simulink model "V40AeroDynamics_edit_3D"  (R2017b)
settings: Solver=VariableStepAuto  StartTime=0.0  StopTime=500  RelTol=1e-3
values from neighbouring files (symbols this model uses):
  A = [ 0        0        0        1 ... (first row only)    [LinearV40.m]
  B = [ 0         0 ... (first row only)    [LinearV40.m]
  b_ref = 5.1    [V40_CFD.mat]
  C = [1       0       0       0 ... (first row only)    [LinearV40.m]
  c_bar = 0.321    [V40_CFD.mat]
  CG_ref_x = 1.38    [V40_CFD.mat]
  CG_ref_z = 0    [V40_CFD.mat]
  CL0 = 0.3831    [V40_CFD.mat]
  Clp = -0.595    [V40_CFD.mat]
  Clr = 0.005    [V40_CFD.mat]
  Cm0 = 0.109    [V40_CFD.mat]
  Cmq = -24.09    [V40_CFD.mat]
  Cnp = 0    [V40_CFD.mat]
  Cnr = -0.023    [V40_CFD.mat]
  CX_d_ca_l =     [V40_CFD.mat]
  CX_d_ca_r =     [V40_CFD.mat]
  CX_d_ea_l =     [V40_CFD.mat]
  CX_d_ea_r =     [V40_CFD.mat]
  CX_d_r =     [V40_CFD.mat]
  D = zeros(size(C,1),2)    [LinearV40.m]
  D_CL_alpha = [-1.0711 -0.8677 -0.6557 -0.4384 -0.2189 0 0.2148 0.422 0.6186 0.8018 0.9688 1.1173 ... (17 elements, 1x17)]    [V40_CFD.mat]
  D_Cm_alpha = [0.0153 0.0193 0.0198 0.0168 0.0102 0 -0.0133 -0.0293 -0.0475 -0.0672 -0.0875 -0.1073 ... (17 elements, 1x17)]    [V40_CFD.mat]
  DCD_alpha = [0.1342 0.0942 0.065 0.0469 0.0395 0.0429 0.0567 0.0807 0.1143 0.1571 0.2086 0.2683 ... (17 elements, 1x17)]    [V40_CFD.mat]
  DCX_beta =     [V40_CFD.mat]
  g = 9.79    [trim_v40.m]    (also in trim_v40_3D.m = 9.8)
  Iv = [13.1154, 0, 0; 0, 9.9543, 0; 0, 0, 15.7149]    [trim_v40.m]    (also in trim_v40_3D.m)
  pitchTheta0 = 0.0521    [LinearV40.m]
  q0 = 0    [LinearV40.m]    (also in trim_v40.m; trim_v40_3D.m)
  rho = 1.213    [trim_v40.m]    (also in trim_v40_3D.m)
  S_ref = 1.4    [V40_CFD.mat]
  Thrust = 39.9    [LinearV40.m]    (also in trim_v40_3D.m = 64.7)
  u0 = 26.152    [LinearV40.m]    (also in trim_v40.m = Vg(1); trim_v40_3D.m = Vg(1))
  w0 = 1.231    [LinearV40.m]    (also in trim_v40.m = Vg(3); trim_v40_3D.m = Vg(3))
  x0 = 0    [LinearV40.m]    (also in trim_v40.m; trim_v40_3D.m)
  x_CG = 1.38-0.043    (= 1.337)    [trim_v40.m]    (also in trim_v40_3D.m)
  z0 = -200    [LinearV40.m]    (also in trim_v40.m; trim_v40_3D.m)
  z_CG = 0    [trim_v40.m]    (also in trim_v40_3D.m)
libraries: simulink_extras x3, shared3dof x1, aerolibasang x1, aerolibtransform2 x1
(part 1 of 2)
settings Model: Creator=ken  LastModifiedBy=ken

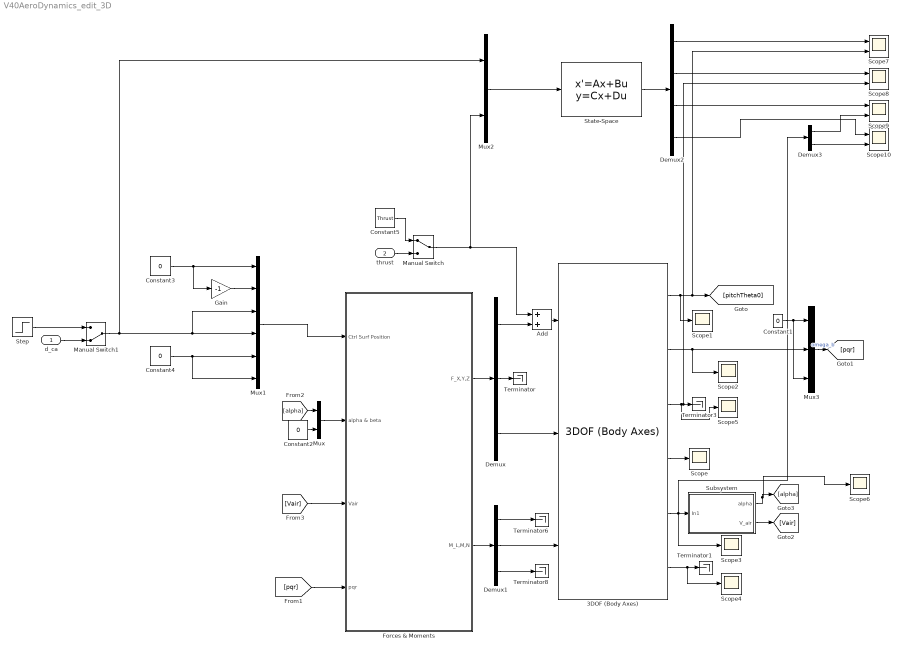
== system V40AeroDynamics_edit_3D ==
  d_ca : Inport
  thrust : Inport  Port=2
  3DOF (Body Axes) : shared3dof/3DOF (Body Axes)  units=Metric (MKS)  mtype=Fixed  v_ini=Vair0  theta_ini=pitchTheta0  alpha_ini=alpha0  q_ini=q0  pos_ini=[x0,z0]  mass=mass0  mass_e=0.5  mass_f=3.0  Iyy=Iv(2,2)  Iyy_e=0.5  Iyy_f=3.0  g_in=Internal  g=g  vre_flag=on  abi_flag=off
      settings: SourceProductName=Aerospace Blockset  SourceProductBaseCode=AE
  Add : Sum
  Constant{1..4} (4 alike) : Constant  Value=0
  Constant5 : Constant  Value=Thrust
  Demux : Demux  Outputs=3
  Demux1 : Demux  Outputs=3
  Demux2 : Demux
  Demux3 : Demux  Outputs=2
  Forces & Moments : Subsystem
  Gain : Gain  Gain=-1
  Manual Switch : ManualSwitch
  Manual Switch1 : ManualSwitch  CurrentSetting=0
  Mux : Mux  Inputs=2
  Mux1 : Mux  Inputs=6
  Mux2 : Mux  Inputs=2
  Mux3 : Mux  Inputs=3
  Scope{,1..6} (7 alike) : Scope
  Scope{7..10} (4 alike) : Scope  NumInputPorts=2
  State-Space : StateSpace  A=A  B=B  C=C  D=D  InitialCondition=[pitchTheta0 u0 w0 q0]
  Step : Step  After=5  SampleTime=0
  Subsystem : Subsystem
  Terminator{,1,3,6,8} (5 alike) : Terminator
  wires:
  Forces & Moments/2(M_L,M,N) -> Demux1/1
  Gain/1 -> Mux1/2
  Constant4/1 -> Mux1/6, Mux1/5
  Demux/2 -> Terminator/1
  Constant3/1 -> Gain/1, Mux1/1
  Demux/3 -> 3DOF (Body Axes)/2
  Manual Switch/1 -> Add/1, Mux2/2
  Demux1/3 -> Terminator8/1
  Demux1/1 -> Terminator6/1
  Forces & Moments/1(F_X,Y,Z) -> Demux/1
  Mux1/1 -> Forces & Moments/1(Ctrl Surf Position)
  Manual Switch1/1 -> Mux2/1, Mux1/3, Mux1/4
  Constant2/1 -> Mux/2
  Mux/1 -> Forces & Moments/2(alpha & beta)
  3DOF (Body Axes)/4 -> Scope/1
  3DOF (Body Axes)/3 -> Scope5/1, Scope8/2, Terminator3/1
  3DOF (Body Axes)/2 -> Scope2/1, Mux3/2
  Constant1/1 -> Mux3/3, Mux3/1
  3DOF (Body Axes)/6 -> Scope4/1, Terminator1/1
  thrust/1 -> Manual Switch/2
  Constant5/1 -> Manual Switch/1
  d_ca/1 -> Manual Switch1/2
  Step/1 -> Manual Switch1/1
  3DOF (Body Axes)/1 -> Scope1/1, Scope7/2, [pitchTheta0]
  Mux3/1 -> [pqr]  "omega_b"
  [pqr] -> Forces & Moments/4(pqr)
  3DOF (Body Axes)/5 -> Demux3/1, Scope3/1, Subsystem/1(In1)
  Subsystem/2(V_air) -> [Vair]
  Subsystem/1(alpha) -> Scope6/1, [alpha]
  [Vair] -> Forces & Moments/3(Vair)
  [alpha] -> Mux/1
  Demux1/2 -> 3DOF (Body Axes)/3
  Demux/1 -> Add/2
  Add/1 -> 3DOF (Body Axes)/1
  Mux2/1 -> State-Space/1
  State-Space/1 -> Demux2/1
  Demux2/1 -> Scope7/1
  Demux2/2 -> Scope8/1
  Demux2/3 -> Scope9/1
  Demux3/1 -> Scope9/2
  Demux2/4 -> Scope10/1
  Demux3/2 -> Scope10/2

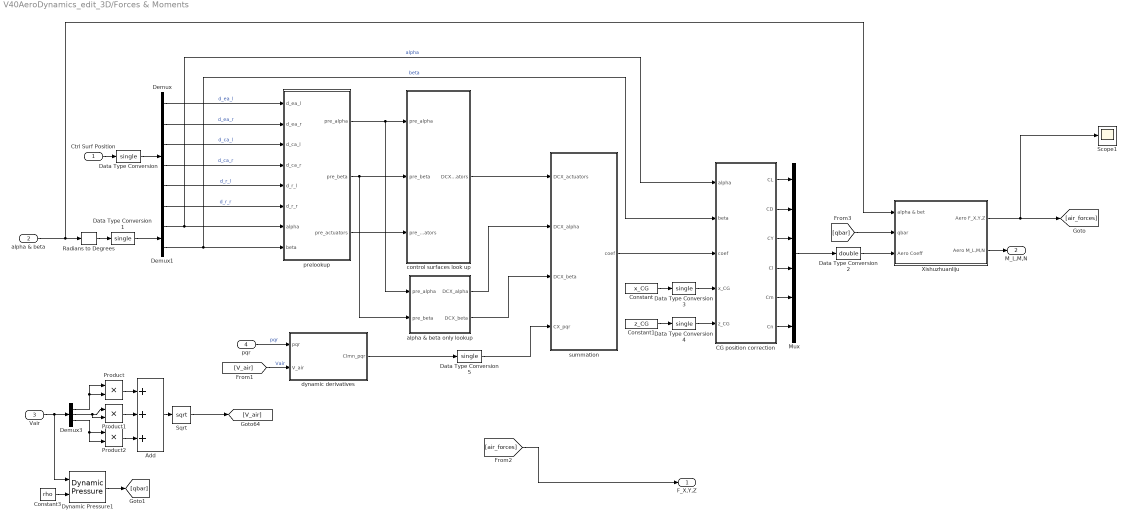
== system V40AeroDynamics_edit_3D/Forces & Moments ==
  Ctrl Surf Position : Inport
  alpha & beta : Inport  Port=2
  Vair : Inport  Port=3
  pqr : Inport  Port=4
  Add : Sum  Inputs=+++
  CG position correction : Subsystem
  Constant : Constant  Value=x_CG
  Constant1 : Constant  Value=z_CG
  Constant3 : Constant  Value=rho
  Data Type Conversion{,1,3..5} (5 alike) : DataTypeConversion  OutDataTypeStr=single
  Data Type Conversion2 : DataTypeConversion  OutDataTypeStr=double
  Demux : Demux  Outputs=6
  Demux1 : Demux  Outputs=2
  Demux3 : Demux  Outputs=3
  Dynamic Pressure1 : aerolibasang/Dynamic Pressure
  Mux : Mux  Inputs=6
  Product : Product
  Product1 : Product
  Product2 : Product
  Radians to Degrees : simulink_extras/Transformations/Radians to Degrees
  Scope1 : Scope
  Sqrt : Sqrt  SaturateOnIntegerOverflow=on
  Xishuzhuanliju : Subsystem
  alpha & beta only lookup : Subsystem
  control surfaces look up : Subsystem
  dynamic derivatives : Subsystem
  prelookup : Subsystem
  summation : Subsystem
  F_X,Y,Z : Outport
  M_L,M,N : Outport  Port=2
  wires:
  Xishuzhuanliju/1(Aero F_X,Y,Z) -> Scope1/1, [air_forces]
  [qbar] -> Xishuzhuanliju/2(qbar)
  Ctrl Surf Position/1 -> Data Type Conversion/1
  alpha & beta/1 -> Xishuzhuanliju/1(alpha & bet), Radians to Degrees/1
  Mux/1 -> Data Type Conversion2/1
  Xishuzhuanliju/2(Aero M_L,M,N) -> M_L,M,N/1
  Vair/1 -> Dynamic Pressure1/1, Demux3/1
  Demux3/1 -> Product/2, Product/1
  Product/1 -> Add/1
  Demux3/3 -> Product2/2, Product2/1
  Product2/1 -> Add/3
  Add/1 -> Sqrt/1
  Demux3/2 -> Product1/2, Product1/1
  Sqrt/1 -> [V_air]
  Product1/1 -> Add/2
  [air_forces] -> F_X,Y,Z/1
  Constant3/1 -> Dynamic Pressure1/2
  Dynamic Pressure1/1 -> [qbar]
  CG position correction/4(Cl) -> Mux/4
  Demux1/1 -> prelookup/7(alpha), CG position correction/1(alpha)  "alpha"
  summation/1(coef) -> CG position correction/3(coef)
  pqr/1 -> dynamic derivatives/1(pqr)  "pqr"
  alpha & beta only lookup/2(DCX_beta) -> summation/3(DCX_beta)
  Demux/4 -> prelookup/4(d_ca_r)  "d_ca_r"
  prelookup/3(pre_actuators) -> control surfaces look up/3(pre_actuators)
  dynamic derivatives/1(Clmn_pqr) -> Data Type Conversion5/1
  CG position correction/1(CL) -> Mux/1
  Demux/3 -> prelookup/3(d_ca_l)  "d_ca_l"
  CG position correction/3(CY) -> Mux/3
  Demux/5 -> prelookup/5(d_r_l)  "d_r_l"
  [V_air] -> dynamic derivatives/2(V_air)  "Vair"
  prelookup/2(pre_beta) -> alpha & beta only lookup/2(pre_beta), control surfaces look up/2(pre_beta)
  CG position correction/6(Cn) -> Mux/6
  CG position correction/2(CD) -> Mux/2
  Demux/6 -> prelookup/6(d_r_r)  "d_r_r"
  Demux1/2 -> prelookup/8(beta), CG position correction/2(beta)  "beta"
  Constant/1 -> Data Type Conversion3/1
  control surfaces look up/1(DCX_actuators) -> summation/1(DCX_actuators)
  CG position correction/5(Cm) -> Mux/5
  Demux/2 -> prelookup/2(d_ea_r)  "d_ea_r"
  prelookup/1(pre_alpha) -> alpha & beta only lookup/1(pre_alpha), control surfaces look up/1(pre_alpha)
  Constant1/1 -> Data Type Conversion4/1
  Demux/1 -> prelookup/1(d_ea_l)  "d_ea_l"
  alpha & beta only lookup/1(DCX_alpha) -> summation/2(DCX_alpha)
  Radians to Degrees/1 -> Data Type Conversion1/1
  Data Type Conversion/1 -> Demux/1
  Data Type Conversion1/1 -> Demux1/1
  Data Type Conversion2/1 -> Xishuzhuanliju/3(Aero Coeff)
  Data Type Conversion3/1 -> CG position correction/4(x_CG)
  Data Type Conversion4/1 -> CG position correction/5(z_CG)
  Data Type Conversion5/1 -> summation/4(CX_pqr)

== system V40AeroDynamics_edit_3D/Subsystem ==
  In1 : Inport
  Atan2 : Trigonometry  Operator=atan2
  Constant : Constant  Value=0
  Demux2 : Demux  Outputs=2
  Mux2 : Mux  Inputs=3
  alpha : Outport
  V_air : Outport  Port=2
  wires:
  Atan2/1 -> alpha/1
  In1/1 -> Demux2/1
  Demux2/2 -> Mux2/3, Atan2/1
  Demux2/1 -> Mux2/1, Atan2/2
  Constant/1 -> Mux2/2
  Mux2/1 -> V_air/1  "V_b"

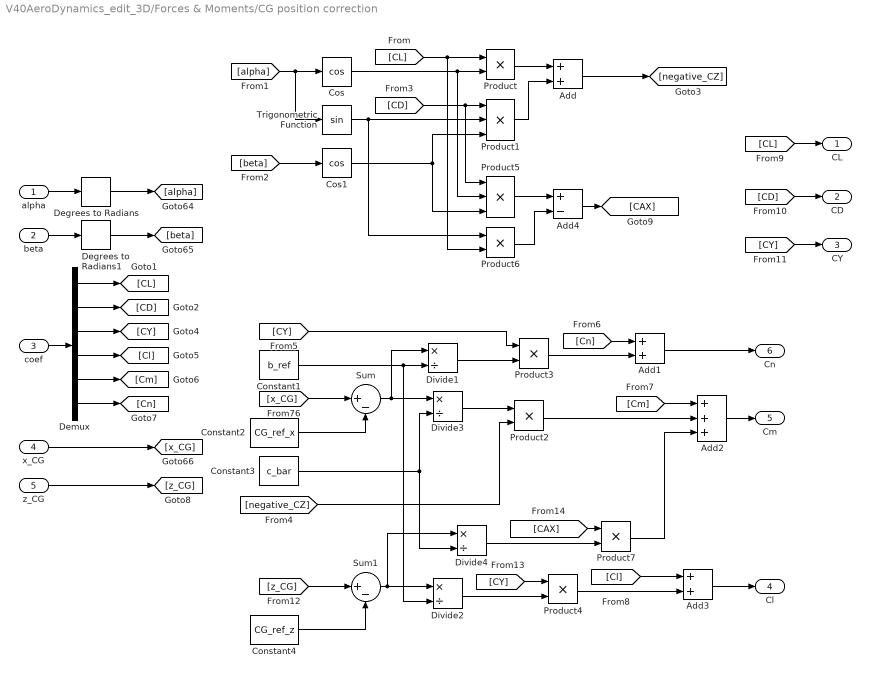
== system V40AeroDynamics_edit_3D/Forces & Moments/CG position correction ==
  alpha : Inport
  beta : Inport  Port=2
  coef : Inport  Port=3
  x_CG : Inport  Port=4
  z_CG : Inport  Port=5
  Add : Sum
  Add1 : Sum
  Add2 : Sum  Inputs=+++
  Add3 : Sum
  Add4 : Sum  Inputs=+-
  Constant1 : Constant  Value=b_ref  OutDataTypeStr=single
  Constant2 : Constant  Value=CG_ref_x  OutDataTypeStr=single
  Constant3 : Constant  Value=c_bar  OutDataTypeStr=single
  Constant4 : Constant  Value=CG_ref_z  OutDataTypeStr=single
  Cos : Trigonometry  Operator=cos
  Cos1 : Trigonometry  Operator=cos
  Degrees to Radians : simulink_extras/Transformations/Degrees to Radians
  Degrees to Radians1 : simulink_extras/Transformations/Degrees to Radians
  Demux : Demux  Outputs=6
  Divide{1..4} (4 alike) : Product  Inputs=*/
  Product{,2..4,6..7} (6 alike) : Product
  Product1 : Product  Inputs=3
  Product5 : Product  Inputs=3
  Sum : Sum  Inputs=|+-
  Sum1 : Sum  Inputs=|+-  OutDataTypeStr=single
  Trigonometric Function : Trigonometry
  CL : Outport
  CD : Outport  Port=2
  CY : Outport  Port=3
  Cl : Outport  Port=4
  Cm : Outport  Port=5
  Cn : Outport  Port=6
  wires:
  x_CG/1 -> [x_CG]
  beta/1 -> Degrees to Radians1/1
  Sum/1 -> Divide1/1, Divide3/1
  Constant3/1 -> Divide4/2, Divide3/2
  alpha/1 -> Degrees to Radians/1
  [alpha] -> Trigonometric Function/1, Cos/1
  [beta] -> Cos1/1
  [CL] -> Product6/2, Product/1
  Cos/1 -> Product5/2, Product/2
  Trigonometric Function/1 -> Product1/2, Product6/1
  [CD] -> Product5/1, Product1/1
  Cos1/1 -> Product5/3, Product1/3
  Product/1 -> Add/1
  Product1/1 -> Add/2
  Add/1 -> [negative_CZ]
  [x_CG] -> Sum/1
  Constant2/1 -> Sum/2
  Divide3/1 -> Product2/1
  [negative_CZ] -> Product2/2
  Divide1/1 -> Product3/2
  Constant1/1 -> Divide2/2, Divide1/2
  [CY] -> Product3/1
  coef/1 -> Demux/1
  Demux/1 -> [CL]
  Demux/2 -> [CD]
  Demux/3 -> [CY]
  Demux/4 -> [Cl]
  Demux/5 -> [Cm]
  Demux/6 -> [Cn]
  Product3/1 -> Add1/2
  [Cn] -> Add1/1
  Product2/1 -> Add2/2
  [Cm] -> Add2/1
  [CL] -> CL/1
  [CD] -> CD/1
  [CY] -> CY/1
  Add3/1 -> Cl/1
  Add1/1 -> Cn/1
  Add2/1 -> Cm/1
  z_CG/1 -> [z_CG]
  [z_CG] -> Sum1/1
  Constant4/1 -> Sum1/2
  Sum1/1 -> Divide2/1, Divide4/1
  Divide2/1 -> Product4/2
  [CY] -> Product4/1
  Product4/1 -> Add3/2
  [Cl] -> Add3/1
  Product5/1 -> Add4/1
  Product6/1 -> Add4/2
  Add4/1 -> [CAX]
  Divide4/1 -> Product7/2
  [CAX] -> Product7/1
  Product7/1 -> Add2/3
  Degrees to Radians/1 -> [alpha]
  Degrees to Radians1/1 -> [beta]

== system V40AeroDynamics_edit_3D/Forces & Moments/Xishuzhuanliju ==
  alpha & bet : Inport
  qbar : Inport  Port=2
  Aero Coeff : Inport  Port=3
  Constant : Constant  Value=[b_ref, c_bar, b_ref]
  Demux : Demux  Outputs=3
  Demux3 : Demux  Outputs=[3,3]
  Demux4 : Demux  Outputs=3
  Direction Cosine Matrix Body to Wind1 : aerolibtransform2/Direction Cosine Matrix Body to Wind
      settings: SourceProductName=Aerospace Blockset  SourceProductBaseCode=AE
  Gain : Gain  Gain=-1
  Gain1 : Gain  Gain=-1
  Mux1 : Mux  Inputs=3
  Mux3 : Mux  Inputs=3
  Product1 : Product  SaturateOnIntegerOverflow=on  InputSameDT=on  OutDataTypeStr=Inherit: Same as first input
  Product4 : Product  SaturateOnIntegerOverflow=on  InputSameDT=on  OutDataTypeStr=Inherit: Same as first input
  Product5 : Product  Multiplication=Matrix(*)  SaturateOnIntegerOverflow=on  InputSameDT=on  OutDataTypeStr=Inherit: Same as first input
  Terminator : Terminator
  Transpose1 : Math  Operator=transpose  SaturateOnIntegerOverflow=on
  Virtual CY : Constant  Value=0
  r : Gain  Gain=S_ref  SaturateOnIntegerOverflow=on  OutDataTypeStr=Inherit: Same as input  ParamDataTypeStr=Inherit: Same as input
  Aero F_X,Y,Z : Outport
  Aero M_L,M,N : Outport  Port=2
  wires:
  Constant/1 -> Product1/2
  Product1/1 -> Aero M_L,M,N/1
  Demux4/3 -> [FY]
  alpha & bet/1 -> Direction Cosine Matrix Body to Wind1/1
  [Drag] -> Gain1/1
  Gain1/1 -> Mux3/1
  Product5/1 -> Demux/1
  Virtual CY/1 -> Mux3/2
  Demux3/1 -> Demux4/1
  Product4/1 -> Demux3/1
  Mux3/1 -> Product5/2
  Transpose1/1 -> Product5/1
  Demux3/2 -> Product1/1
  Mux1/1 -> Aero F_X,Y,Z/1
  Direction Cosine Matrix Body to Wind1/1 -> Transpose1/1
  qbar/1 -> r/1
  Demux/1 -> Mux1/1
  Demux/3 -> Mux1/3
  [FY] -> Mux1/2
  Demux/2 -> Terminator/1
  Demux4/1 -> [Lift]
  Demux4/2 -> [Drag]
  Gain/1 -> Mux3/3
  [Lift] -> Gain/1
  r/1 -> Product4/1
  Aero Coeff/1 -> Product4/2

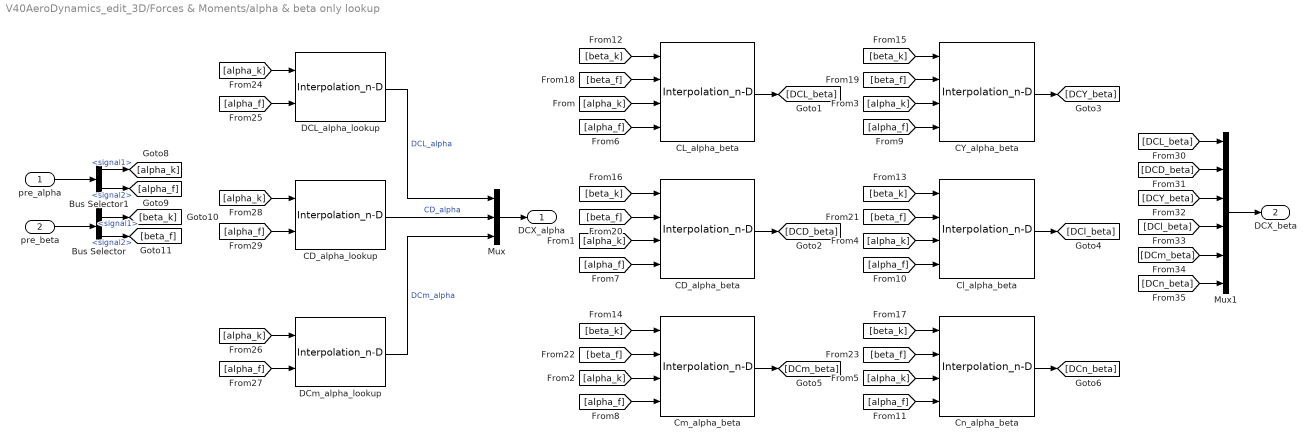
== system V40AeroDynamics_edit_3D/Forces & Moments/alpha & beta only lookup ==
  pre_alpha : Inport
  pre_beta : Inport  Port=2
  Bus Selector : BusSelector  OutputSignals=signal1,signal2
  Bus Selector1 : BusSelector  OutputSignals=signal1,signal2
  CD_alpha_beta : Interpolation_n-D  Table=DCX_beta{2}  OutDataTypeStr=single
  CD_alpha_lookup : Interpolation_n-D  NumberOfTableDimensions=1  Table=DCD_alpha  OutDataTypeStr=single
      settings: InputPortMap=u0,u1
  CL_alpha_beta : Interpolation_n-D  Table=DCX_beta{1}  OutDataTypeStr=single
  CY_alpha_beta : Interpolation_n-D  Table=DCX_beta{4}  OutDataTypeStr=single
  Cl_alpha_beta : Interpolation_n-D  Table=DCX_beta{6}  OutDataTypeStr=single
  Cm_alpha_beta : Interpolation_n-D  Table=DCX_beta{3}  OutDataTypeStr=single
  Cn_alpha_beta : Interpolation_n-D  Table=DCX_beta{5}  OutDataTypeStr=single
  DCL_alpha_lookup : Interpolation_n-D  NumberOfTableDimensions=1  Table=D_CL_alpha  OutDataTypeStr=single
      settings: InputPortMap=u0,u1
  DCm_alpha_lookup : Interpolation_n-D  NumberOfTableDimensions=1  Table=D_Cm_alpha  OutDataTypeStr=single
      settings: InputPortMap=u0,u1
  Mux : Mux  Inputs=3
  Mux1 : Mux  Inputs=6
  DCX_alpha : Outport
  DCX_beta : Outport  Port=2
  wires:
  pre_alpha/1 -> Bus Selector1/1
  pre_beta/1 -> Bus Selector/1
  Bus Selector1/2 -> [alpha_f]  "<signal2>"
  Bus Selector/1 -> [beta_k]  "<signal1>"
  Bus Selector/2 -> [beta_f]  "<signal2>"
  Bus Selector1/1 -> [alpha_k]  "<signal1>"
  CL_alpha_beta/1 -> [DCL_beta]
  Cn_alpha_beta/1 -> [DCn_beta]
  Cl_alpha_beta/1 -> [DCl_beta]
  CY_alpha_beta/1 -> [DCY_beta]
  CD_alpha_beta/1 -> [DCD_beta]
  Cm_alpha_beta/1 -> [DCm_beta]
  [beta_k] -> CL_alpha_beta/1
  [beta_f] -> CL_alpha_beta/2
  [alpha_k] -> CL_alpha_beta/3
  [alpha_f] -> CL_alpha_beta/4
  [beta_k] -> CY_alpha_beta/1
  [beta_f] -> CY_alpha_beta/2
  [alpha_k] -> CY_alpha_beta/3
  [alpha_f] -> CY_alpha_beta/4
  [beta_k] -> Cl_alpha_beta/1
  [beta_f] -> Cl_alpha_beta/2
  [alpha_k] -> Cl_alpha_beta/3
  [alpha_f] -> Cl_alpha_beta/4
  [beta_k] -> CD_alpha_beta/1
  [beta_f] -> CD_alpha_beta/2
  [alpha_k] -> CD_alpha_beta/3
  [alpha_f] -> CD_alpha_beta/4
  [beta_k] -> Cm_alpha_beta/1
  [beta_f] -> Cm_alpha_beta/2
  [alpha_k] -> Cm_alpha_beta/3
  [alpha_f] -> Cm_alpha_beta/4
  [beta_k] -> Cn_alpha_beta/1
  [beta_f] -> Cn_alpha_beta/2
  [alpha_k] -> Cn_alpha_beta/3
  [alpha_f] -> Cn_alpha_beta/4
  [alpha_k] -> DCL_alpha_lookup/1
  [alpha_f] -> DCL_alpha_lookup/2
  DCL_alpha_lookup/1 -> Mux/1  "DCL_alpha"
  [alpha_k] -> DCm_alpha_lookup/1
  DCm_alpha_lookup/1 -> Mux/3  "DCm_alpha"
  [alpha_f] -> DCm_alpha_lookup/2
  [alpha_k] -> CD_alpha_lookup/1
  CD_alpha_lookup/1 -> Mux/2  "CD_alpha"
  [alpha_f] -> CD_alpha_lookup/2
  Mux/1 -> DCX_alpha/1
  [DCL_beta] -> Mux1/1
  [DCD_beta] -> Mux1/2
  [DCY_beta] -> Mux1/3
  [DCl_beta] -> Mux1/4
  [DCm_beta] -> Mux1/5
  [DCn_beta] -> Mux1/6
  Mux1/1 -> DCX_beta/1

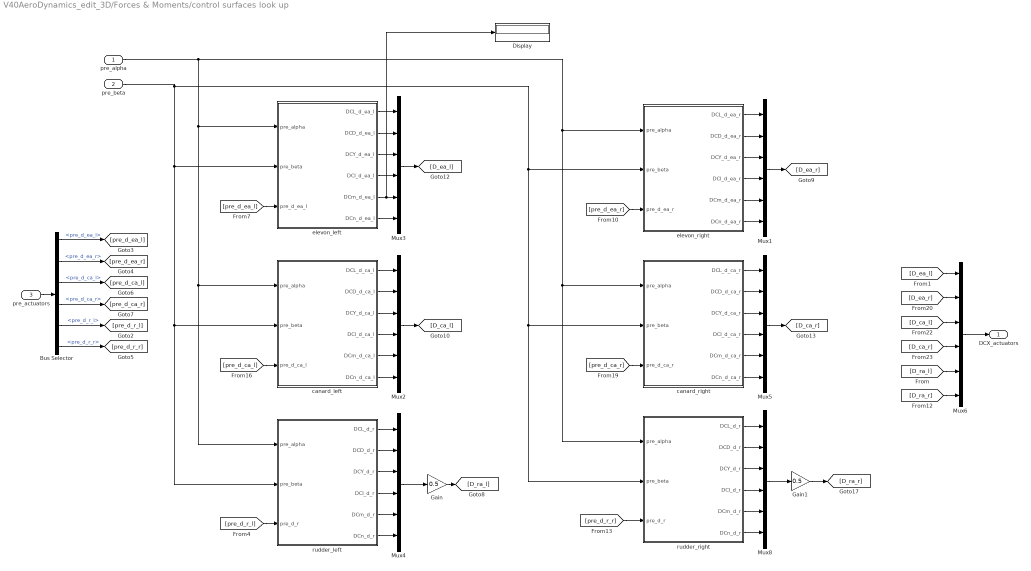
== system V40AeroDynamics_edit_3D/Forces & Moments/control surfaces look up ==
  pre_alpha : Inport
  pre_beta : Inport  Port=2
  pre_actuators : Inport  Port=3
  Bus Selector : BusSelector  OutputSignals=pre_d_ea_l,pre_d_ea_r,pre_d_ca_l,pre_d_ca_r,pre_d_r_l,pre_d_r_r
  Display : Display
  Gain : Gain  Gain=0.5
  Gain1 : Gain  Gain=0.5
  Mux{1..6,8} (7 alike) : Mux  Inputs=6
  canard_left : Subsystem
  canard_right : Subsystem
  "elevon_left " : Subsystem
  "elevon_right " : Subsystem
  rudder_left : Subsystem
  rudder_right : Subsystem
  DCX_actuators : Outport
  wires:
  "elevon_right "/6(DCn_d_ea_r) -> Mux1/6
  "elevon_right "/5(DCm_d_ea_r) -> Mux1/5
  "elevon_right "/1(DCL_d_ea_r) -> Mux1/1
  [pre_d_ea_l] -> "elevon_left "/3(pre_d_ea_l)
  "elevon_left "/2(DCD_d_ea_l) -> Mux3/2
  canard_right/3(DCY_d_ca_r) -> Mux5/3
  "elevon_left "/1(DCL_d_ea_l) -> Mux3/1
  canard_left/5(DCm_d_ca_l) -> Mux2/5
  canard_left/4(DCl_d_ca_l) -> Mux2/4
  "elevon_right "/3(DCY_d_ea_r) -> Mux1/3
  canard_left/3(DCY_d_ca_l) -> Mux2/3
  "elevon_right "/4(DCl_d_ea_r) -> Mux1/4
  "elevon_left "/5(DCm_d_ea_l) -> Display/1, Mux3/5
  "elevon_left "/3(DCY_d_ea_l) -> Mux3/3
  canard_right/2(DCD_d_ca_r) -> Mux5/2
  canard_left/6(DCn_d_ca_l) -> Mux2/6
  "elevon_left "/6(DCn_d_ea_l) -> Mux3/6
  "elevon_left "/4(DCl_d_ea_l) -> Mux3/4
  canard_right/6(DCn_d_ca_r) -> Mux5/6
  canard_left/1(DCL_d_ca_l) -> Mux2/1
  canard_right/5(DCm_d_ca_r) -> Mux5/5
  canard_left/2(DCD_d_ca_l) -> Mux2/2
  canard_right/1(DCL_d_ca_r) -> Mux5/1
  "elevon_right "/2(DCD_d_ea_r) -> Mux1/2
  canard_right/4(DCl_d_ca_r) -> Mux5/4
  Mux3/1 -> [D_ea_l]
  Mux1/1 -> [D_ea_r]
  Mux2/1 -> [D_ca_l]
  Mux5/1 -> [D_ca_r]
  Bus Selector/1 -> [pre_d_ea_l]  "<pre_d_ea_l>"
  Bus Selector/2 -> [pre_d_ea_r]  "<pre_d_ea_r>"
  Bus Selector/3 -> [pre_d_ca_l]  "<pre_d_ca_l>"
  Mux6/1 -> DCX_actuators/1
  Bus Selector/4 -> [pre_d_ca_r]  "<pre_d_ca_r>"
  pre_actuators/1 -> Bus Selector/1
  [pre_d_ea_r] -> "elevon_right "/3(pre_d_ea_r)
  [pre_d_ca_l] -> canard_left/3(pre_d_ca_l)
  [pre_d_ca_r] -> canard_right/3(pre_d_ca_r)
  rudder_right/3(DCY_d_r) -> Mux8/3
  pre_alpha/1 -> rudder_left/1(pre_alpha), canard_left/1(pre_alpha), "elevon_left "/1(pre_alpha), rudder_right/1(pre_alpha), canard_right/1(pre_alpha), "elevon_right "/1(pre_alpha)
  rudder_right/4(DCl_d_r) -> Mux8/4
  Mux8/1 -> Gain1/1
  rudder_right/2(DCD_d_r) -> Mux8/2
  pre_beta/1 -> canard_left/2(pre_beta), rudder_left/2(pre_beta), "elevon_left "/2(pre_beta), canard_right/2(pre_beta), rudder_right/2(pre_beta), "elevon_right "/2(pre_beta)
  rudder_right/1(DCL_d_r) -> Mux8/1
  rudder_right/6(DCn_d_r) -> Mux8/6
  rudder_right/5(DCm_d_r) -> Mux8/5
  [pre_d_r_r] -> rudder_right/3(pre_d_r)
  rudder_left/1(DCL_d_r) -> Mux4/1
  [pre_d_r_l] -> rudder_left/3(pre_d_r)
  rudder_left/4(DCl_d_r) -> Mux4/4
  rudder_left/6(DCn_d_r) -> Mux4/6
  Mux4/1 -> Gain/1
  rudder_left/5(DCm_d_r) -> Mux4/5
  rudder_left/2(DCD_d_r) -> Mux4/2
  rudder_left/3(DCY_d_r) -> Mux4/3
  [D_ea_l] -> Mux6/1
  [D_ea_r] -> Mux6/2
  [D_ca_l] -> Mux6/3
  [D_ca_r] -> Mux6/4
  [D_ra_l] -> Mux6/5
  [D_ra_r] -> Mux6/6
  Bus Selector/5 -> [pre_d_r_l]  "<pre_d_r_l>"
  Bus Selector/6 -> [pre_d_r_r]  "<pre_d_r_r>"
  Gain/1 -> [D_ra_l]
  Gain1/1 -> [D_ra_r]

== system V40AeroDynamics_edit_3D/Forces & Moments/dynamic derivatives ==
  pqr : Inport
  V_air : Inport  Port=2
  Add : Sum
  Add1 : Sum
  Demux : Demux  Outputs=3
  Divide : Product  Inputs=*/  OutDataTypeStr=double
  Divide1 : Product  Inputs=*/  OutDataTypeStr=double
  Divide2 : Product  Inputs=*/  OutDataTypeStr=double
  Gain : Gain  Gain=Cmq
  Gain1 : Gain  Gain=b_ref
  Gain10 : Gain  Gain=0.5
  Gain2 : Gain  Gain=Clp
  Gain3 : Gain  Gain=Clr
  Gain4 : Gain  Gain=b_ref
  Gain5 : Gain  Gain=Cnp
  Gain6 : Gain  Gain=Cnr
  Gain7 : Gain  Gain=0.5
  Gain8 : Gain  Gain=0.5
  Gain9 : Gain  Gain=c_bar
  Mux : Mux  Inputs=3
  Clmn_pqr : Outport
  wires:
  pqr/1 -> Demux/1
  Gain/1 -> Gain9/1
  V_air/1 -> [V_air]
  Demux/2 -> Gain/1
  [V_air] -> Divide/2
  Divide/1 -> Mux/2
  Add/1 -> Gain1/1
  [V_air] -> Divide1/2
  Gain1/1 -> Gain7/1
  Gain2/1 -> Add/1
  Gain3/1 -> Add/2
  Divide1/1 -> Mux/1
  Gain5/1 -> Add1/1
  Demux/1 -> Gain5/1, Gain2/1
  Demux/3 -> Gain3/1, Gain6/1
  Gain4/1 -> Gain10/1
  Add1/1 -> Gain4/1
  [V_air] -> Divide2/2
  Gain6/1 -> Add1/2
  Divide2/1 -> Mux/3
  Gain7/1 -> Divide1/1
  Gain8/1 -> Divide/1
  Gain9/1 -> Gain8/1
  Gain10/1 -> Divide2/1
  Mux/1 -> Clmn_pqr/1

== system V40AeroDynamics_edit_3D/Forces & Moments/prelookup ==
  d_ea_l : Inport
  d_ea_r : Inport  Port=2
  d_ca_l : Inport  Port=3
  d_ca_r : Inport  Port=4
  d_r_l : Inport  Port=5
  d_r_r : Inport  Port=6
  alpha : Inport  Port=7
  beta : Inport  Port=8
  Bus Creator{,1..4,6..7,10} (8 alike) : BusCreator  Inputs=2
  Bus Creator8 : BusCreator  Inputs=6
  alpha prelookup : PreLookup  BreakpointsData=alpha_breakpoints  BeginIndexSearchUsingPreviousIndexResult=on  ExtrapMethod=Linear  UseLastBreakpoint=on
  beta prelookup : PreLookup  BreakpointsData=beta_breakpoints  BeginIndexSearchUsingPreviousIndexResult=on  ExtrapMethod=Linear  UseLastBreakpoint=on
  d_ca_l prelookup : PreLookup  BreakpointsData=delta_breakpoints  BeginIndexSearchUsingPreviousIndexResult=on  ExtrapMethod=Linear  UseLastBreakpoint=on
  d_ca_r prelookup : PreLookup  BreakpointsData=delta_breakpoints  BeginIndexSearchUsingPreviousIndexResult=on  ExtrapMethod=Linear  UseLastBreakpoint=on
  d_ea_l prelookup : PreLookup  BreakpointsData=delta_breakpoints  BeginIndexSearchUsingPreviousIndexResult=on  ExtrapMethod=Linear  UseLastBreakpoint=on
  d_ea_r prelookup : PreLookup  BreakpointsData=delta_breakpoints  BeginIndexSearchUsingPreviousIndexResult=on  ExtrapMethod=Linear  UseLastBreakpoint=on
  d_r_l prelookup : PreLookup  BreakpointsData=delta_breakpoints  BeginIndexSearchUsingPreviousIndexResult=on  ExtrapMethod=Linear  UseLastBreakpoint=on
  d_r_r prelookup1 : PreLookup  BreakpointsData=delta_breakpoints  BeginIndexSearchUsingPreviousIndexResult=on  ExtrapMethod=Linear  UseLastBreakpoint=on
  pre_alpha : Outport
  pre_beta : Outport  Port=2
  pre_actuators : Outport  Port=3
  wires:
  beta prelookup/2 -> Bus Creator1/2
  d_ea_r prelookup/1 -> Bus Creator4/1
  alpha prelookup/1 -> Bus Creator/1
  alpha prelookup/2 -> Bus Creator/2
  d_ca_l prelookup/1 -> Bus Creator6/1
  d_ea_r prelookup/2 -> Bus Creator4/2
  Bus Creator1/1 -> pre_beta/1
  Bus Creator/1 -> pre_alpha/1
  alpha/1 -> alpha prelookup/1
  d_ea_l prelookup/1 -> Bus Creator3/1
  d_ea_l prelookup/2 -> Bus Creator3/2
  d_ea_r/1 -> d_ea_r prelookup/1
  d_ca_l/1 -> d_ca_l prelookup/1
  d_ea_l/1 -> d_ea_l prelookup/1
  beta prelookup/1 -> Bus Creator1/1
  d_ca_l prelookup/2 -> Bus Creator6/2
  beta/1 -> beta prelookup/1
  d_ca_r prelookup/1 -> Bus Creator7/1
  d_ca_r prelookup/2 -> Bus Creator7/2
  d_ca_r/1 -> d_ca_r prelookup/1
  Bus Creator3/1 -> Bus Creator8/1  "pre_d_ea_l"
  Bus Creator4/1 -> Bus Creator8/2  "pre_d_ea_r"
  Bus Creator6/1 -> Bus Creator8/3  "pre_d_ca_l"
  Bus Creator7/1 -> Bus Creator8/4  "pre_d_ca_r"
  Bus Creator8/1 -> pre_actuators/1
  d_r_l/1 -> d_r_l prelookup/1
  d_r_l prelookup/1 -> Bus Creator10/1
  d_r_l prelookup/2 -> Bus Creator10/2
  Bus Creator10/1 -> Bus Creator8/5  "pre_d_r_l"
  d_r_r/1 -> d_r_r prelookup1/1
  d_r_r prelookup1/1 -> Bus Creator2/1
  Bus Creator2/1 -> Bus Creator8/6  "pre_d_r_r"
  d_r_r prelookup1/2 -> Bus Creator2/2

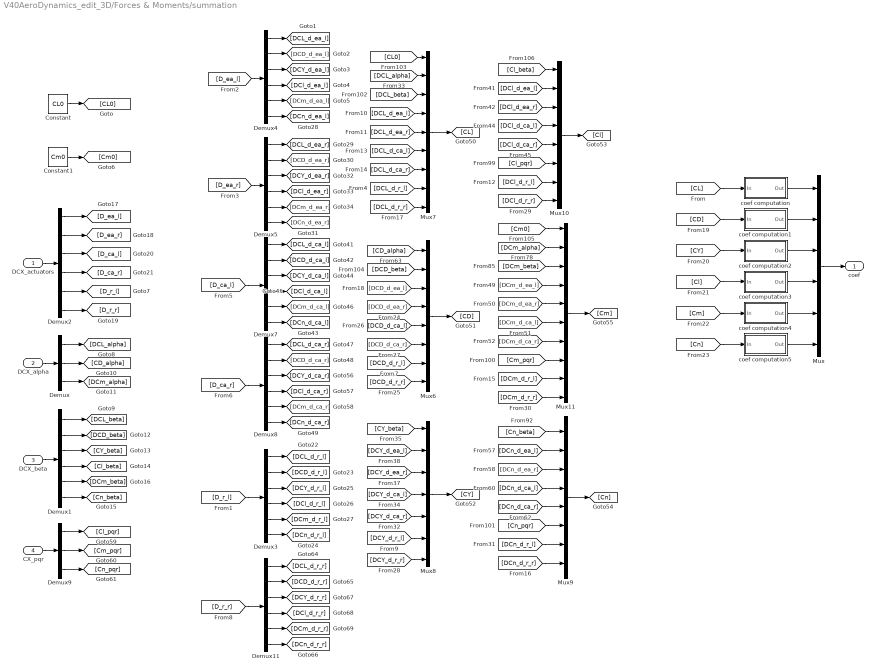
== system V40AeroDynamics_edit_3D/Forces & Moments/summation ==
  DCX_actuators : Inport
  DCX_alpha : Inport  Port=2
  DCX_beta : Inport  Port=3
  CX_pqr : Inport  Port=4
  Constant : Constant  Value=CL0  OutDataTypeStr=single
  Constant1 : Constant  Value=Cm0  OutDataTypeStr=single
  Demux : Demux  Outputs=3
  Demux{1..5,7..8,11} (8 alike) : Demux  Outputs=6
  Demux9 : Demux  Outputs=3
  Mux : Mux  Inputs=6
  Mux10 : Mux  Inputs=8
  Mux11 : Mux  Inputs=10
  Mux6 : Mux  Inputs=8
  Mux7 : Mux  Inputs=9
  Mux8 : Mux  Inputs=7
  Mux9 : Mux  Inputs=8
  coef computation : Subsystem
  coef computation1 : Subsystem
  coef computation2 : Subsystem
  coef computation3 : Subsystem
  coef computation4 : Subsystem
  coef computation5 : Subsystem
  coef : Outport
  wires:
  DCX_actuators/1 -> Demux2/1
  DCX_alpha/1 -> Demux/1
  DCX_beta/1 -> Demux1/1
  Demux/1 -> [DCL_alpha]
  Demux/2 -> [CD_alpha]
  Demux/3 -> [DCm_alpha]
  Demux1/1 -> [DCL_beta]
  Demux1/2 -> [DCD_beta]
  Demux1/3 -> [CY_beta]
  Demux1/4 -> [Cl_beta]
  Demux1/5 -> [DCm_beta]
  Demux1/6 -> [Cn_beta]
  [CL] -> coef computation/1(In)
  [CD] -> coef computation1/1(In)
  [CY] -> coef computation2/1(In)
  [Cl] -> coef computation3/1(In)
  [Cm] -> coef computation4/1(In)
  [Cn] -> coef computation5/1(In)
  coef computation/1(Out) -> Mux/1
  coef computation1/1(Out) -> Mux/2
  coef computation2/1(Out) -> Mux/3
  coef computation3/1(Out) -> Mux/4
  coef computation4/1(Out) -> Mux/5
  coef computation5/1(Out) -> Mux/6
  Mux6/1 -> [CD]
  Mux9/1 -> [Cn]
  Mux11/1 -> [Cm]
  Mux10/1 -> [Cl]
  Mux8/1 -> [CY]
  Mux7/1 -> [CL]
  Demux4/4 -> [DCl_d_ea_l]
  [D_ea_l] -> Demux4/1
  Demux4/2 -> [DCD_d_ea_l]
  Demux4/6 -> [DCn_d_ea_l]
  Demux4/3 -> [DCY_d_ea_l]
  Demux4/1 -> [DCL_d_ea_l]
  Demux4/5 -> [DCm_d_ea_l]
  [D_ea_r] -> Demux5/1
  Demux5/2 -> [DCD_d_ea_r]
  Demux5/5 -> [DCm_d_ea_r]
  Demux5/6 -> [DCn_d_ea_r]
  Demux5/1 -> [DCL_d_ea_r]
  Demux5/3 -> [DCY_d_ea_r]
  Demux5/4 -> [DCl_d_ea_r]
  Demux7/5 -> [DCm_d_ca_l]
  Demux7/4 -> [DCl_d_ca_l]
  [D_ca_l] -> Demux7/1
  Demux7/3 -> [DCY_d_ca_l]
  Demux7/2 -> [DCD_d_ca_l]
  Demux7/1 -> [DCL_d_ca_l]
  Demux7/6 -> [DCn_d_ca_l]
  Demux8/5 -> [DCm_d_ca_r]
  Demux8/4 -> [DCl_d_ca_r]
  [D_ca_r] -> Demux8/1
  Demux8/3 -> [DCY_d_ca_r]
  Demux8/2 -> [DCD_d_ca_r]
  Demux8/1 -> [DCL_d_ca_r]
  Demux8/6 -> [DCn_d_ca_r]
  CX_pqr/1 -> Demux9/1
  Demux9/1 -> [Cl_pqr]
  Demux9/2 -> [Cm_pqr]
  Demux9/3 -> [Cn_pqr]
  Mux/1 -> coef/1
  Constant/1 -> [CL0]
  Constant1/1 -> [Cm0]
  [D_r_r] -> Demux11/1
  Demux11/1 -> [DCL_d_r_r]
  Demux11/2 -> [DCD_d_r_r]
  Demux11/3 -> [DCY_d_r_r]
  Demux11/4 -> [DCl_d_r_r]
  Demux11/5 -> [DCm_d_r_r]
  Demux11/6 -> [DCn_d_r_r]
  Demux2/1 -> [D_ea_l]
  Demux2/2 -> [D_ea_r]
  Demux2/3 -> [D_ca_l]
  Demux2/4 -> [D_ca_r]
  Demux2/5 -> [D_r_l]
  Demux2/6 -> [D_r_r]
  Demux3/1 -> [DCL_d_r_l]
  Demux3/3 -> [DCY_d_r_l]
  Demux3/5 -> [DCm_d_r_l]
  Demux3/4 -> [DCl_d_r_l]
  Demux3/6 -> [DCn_d_r_l]
  Demux3/2 -> [DCD_d_r_l]
  [D_r_l] -> Demux3/1
  [DCL_beta] -> Mux7/3
  [DCL_alpha] -> Mux7/2
  [CL0] -> Mux7/1
  [DCL_d_ea_l] -> Mux7/4
  [DCL_d_ea_r] -> Mux7/5
  [DCL_d_ca_l] -> Mux7/6
  [DCL_d_ca_r] -> Mux7/7
  [Cl_beta] -> Mux10/1
  [DCl_d_ea_l] -> Mux10/2
  [DCl_d_ea_r] -> Mux10/3
  [DCl_d_ca_l] -> Mux10/4
  [DCl_d_ca_r] -> Mux10/5
  [Cl_pqr] -> Mux10/6
  [CD_alpha] -> Mux6/1
  [DCD_beta] -> Mux6/2
  [DCD_d_ea_l] -> Mux6/3
  [DCD_d_ea_r] -> Mux6/4
  [CY_beta] -> Mux8/1
  [DCY_d_ea_l] -> Mux8/2
  [DCY_d_ea_r] -> Mux8/3
  [DCY_d_ca_l] -> Mux8/4
  [DCY_d_ca_r] -> Mux8/5
  [Cm0] -> Mux11/1
  [DCm_alpha] -> Mux11/2
  [DCm_beta] -> Mux11/3
  [DCm_d_ea_l] -> Mux11/4
  [DCm_d_ea_r] -> Mux11/5
  [DCm_d_ca_l] -> Mux11/6
  [DCm_d_ca_r] -> Mux11/7
  [Cm_pqr] -> Mux11/8
  [Cn_beta] -> Mux9/1
  [DCn_d_ea_l] -> Mux9/2
  [DCn_d_ea_r] -> Mux9/3
  [DCn_d_ca_l] -> Mux9/4
  [DCn_d_ca_r] -> Mux9/5
  [Cn_pqr] -> Mux9/6
  [DCD_d_ca_l] -> Mux6/5
  [DCD_d_ca_r] -> Mux6/6
  [DCL_d_r_l] -> Mux7/8
  [DCD_d_r_l] -> Mux6/7
  [DCY_d_r_l] -> Mux8/6
  [DCl_d_r_l] -> Mux10/7
  [DCm_d_r_l] -> Mux11/9
  [DCm_d_r_r] -> Mux11/10
  [DCL_d_r_r] -> Mux7/9
  [DCD_d_r_r] -> Mux6/8
  [DCY_d_r_r] -> Mux8/7
  [DCl_d_r_r] -> Mux10/8
  [DCn_d_r_r] -> Mux9/8
  [DCn_d_r_l] -> Mux9/7

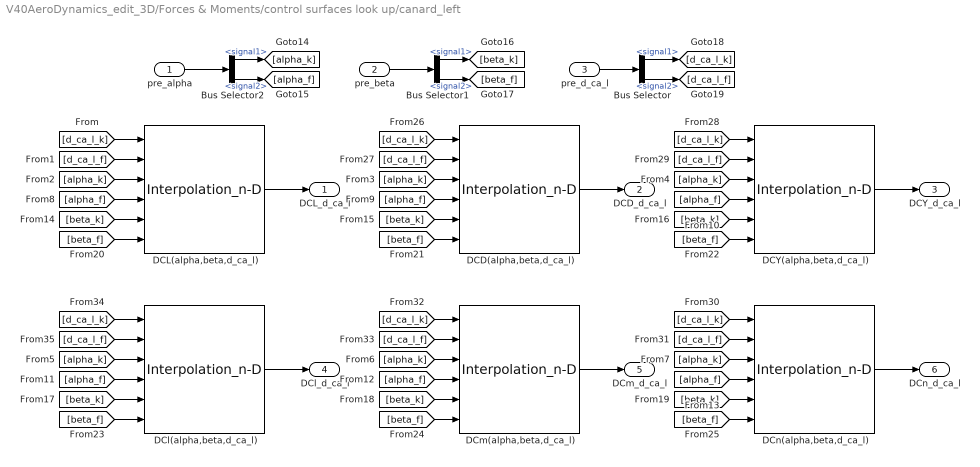
== system V40AeroDynamics_edit_3D/Forces & Moments/control surfaces look up/canard_left ==
  pre_alpha : Inport
  pre_beta : Inport  Port=2
  pre_d_ca_l : Inport  Port=3
  Bus Selector : BusSelector  OutputSignals=signal1,signal2
  Bus Selector1 : BusSelector  OutputSignals=signal1,signal2
  Bus Selector2 : BusSelector  OutputSignals=signal1,signal2
  DCD(alpha,beta,d_ca_l) : Interpolation_n-D  NumberOfTableDimensions=3  Table=CX_d_ca_l{2}  OutDataTypeStr=single
      settings: InputPortMap=u0,u1,u2,u3,u4,u5
  DCL(alpha,beta,d_ca_l) : Interpolation_n-D  NumberOfTableDimensions=3  Table=CX_d_ca_l{1}  OutDataTypeStr=single
      settings: InputPortMap=u0,u1,u2,u3,u4,u5
  DCY(alpha,beta,d_ca_l) : Interpolation_n-D  NumberOfTableDimensions=3  Table=CX_d_ca_l{4}  OutDataTypeStr=single
      settings: InputPortMap=u0,u1,u2,u3,u4,u5
  DCl(alpha,beta,d_ca_l) : Interpolation_n-D  NumberOfTableDimensions=3  Table=CX_d_ca_l{6}  OutDataTypeStr=single
      settings: InputPortMap=u0,u1,u2,u3,u4,u5
  DCm(alpha,beta,d_ca_l) : Interpolation_n-D  NumberOfTableDimensions=3  Table=CX_d_ca_l{3}  OutDataTypeStr=single
      settings: InputPortMap=u0,u1,u2,u3,u4,u5
  DCn(alpha,beta,d_ca_l) : Interpolation_n-D  NumberOfTableDimensions=3  Table=CX_d_ca_l{5}  OutDataTypeStr=single
      settings: InputPortMap=u0,u1,u2,u3,u4,u5
  DCL_d_ca_l : Outport
  DCD_d_ca_l : Outport  Port=2
  DCY_d_ca_l : Outport  Port=3
  DCl_d_ca_l : Outport  Port=4
  DCm_d_ca_l : Outport  Port=5
  DCn_d_ca_l : Outport  Port=6
  wires:
  Bus Selector1/2 -> [beta_f]  "<signal2>"
  DCY(alpha,beta,d_ca_l)/1 -> DCY_d_ca_l/1
  pre_beta/1 -> Bus Selector1/1
  Bus Selector/2 -> [d_ca_l_f]  "<signal2>"
  DCD(alpha,beta,d_ca_l)/1 -> DCD_d_ca_l/1
  DCl(alpha,beta,d_ca_l)/1 -> DCl_d_ca_l/1
  Bus Selector/1 -> [d_ca_l_k]  "<signal1>"
  Bus Selector2/1 -> [alpha_k]  "<signal1>"
  DCm(alpha,beta,d_ca_l)/1 -> DCm_d_ca_l/1
  Bus Selector2/2 -> [alpha_f]  "<signal2>"
  pre_alpha/1 -> Bus Selector2/1
  DCn(alpha,beta,d_ca_l)/1 -> DCn_d_ca_l/1
  DCL(alpha,beta,d_ca_l)/1 -> DCL_d_ca_l/1
  Bus Selector1/1 -> [beta_k]  "<signal1>"
  [beta_k] -> DCL(alpha,beta,d_ca_l)/5
  [beta_f] -> DCL(alpha,beta,d_ca_l)/6
  [beta_k] -> DCD(alpha,beta,d_ca_l)/5
  [beta_f] -> DCD(alpha,beta,d_ca_l)/6
  [beta_k] -> DCY(alpha,beta,d_ca_l)/5
  [beta_f] -> DCY(alpha,beta,d_ca_l)/6
  [beta_k] -> DCl(alpha,beta,d_ca_l)/5
  [beta_f] -> DCl(alpha,beta,d_ca_l)/6
  [beta_k] -> DCm(alpha,beta,d_ca_l)/5
  [beta_f] -> DCm(alpha,beta,d_ca_l)/6
  [beta_k] -> DCn(alpha,beta,d_ca_l)/5
  [beta_f] -> DCn(alpha,beta,d_ca_l)/6
  [d_ca_l_k] -> DCD(alpha,beta,d_ca_l)/1
  [d_ca_l_k] -> DCY(alpha,beta,d_ca_l)/1
  [d_ca_l_k] -> DCn(alpha,beta,d_ca_l)/1
  [d_ca_l_k] -> DCm(alpha,beta,d_ca_l)/1
  [d_ca_l_k] -> DCL(alpha,beta,d_ca_l)/1
  [d_ca_l_f] -> DCL(alpha,beta,d_ca_l)/2
  [alpha_k] -> DCL(alpha,beta,d_ca_l)/3
  [alpha_f] -> DCL(alpha,beta,d_ca_l)/4
  [d_ca_l_k] -> DCl(alpha,beta,d_ca_l)/1
  [d_ca_l_f] -> DCl(alpha,beta,d_ca_l)/2
  [alpha_k] -> DCl(alpha,beta,d_ca_l)/3
  [alpha_f] -> DCl(alpha,beta,d_ca_l)/4
  [d_ca_l_f] -> DCD(alpha,beta,d_ca_l)/2
  [alpha_k] -> DCD(alpha,beta,d_ca_l)/3
  [alpha_f] -> DCD(alpha,beta,d_ca_l)/4
  [d_ca_l_f] -> DCY(alpha,beta,d_ca_l)/2
  [alpha_k] -> DCY(alpha,beta,d_ca_l)/3
  [alpha_f] -> DCY(alpha,beta,d_ca_l)/4
  [d_ca_l_f] -> DCn(alpha,beta,d_ca_l)/2
  [alpha_k] -> DCn(alpha,beta,d_ca_l)/3
  [alpha_f] -> DCn(alpha,beta,d_ca_l)/4
  [d_ca_l_f] -> DCm(alpha,beta,d_ca_l)/2
  [alpha_k] -> DCm(alpha,beta,d_ca_l)/3
  [alpha_f] -> DCm(alpha,beta,d_ca_l)/4
  pre_d_ca_l/1 -> Bus Selector/1

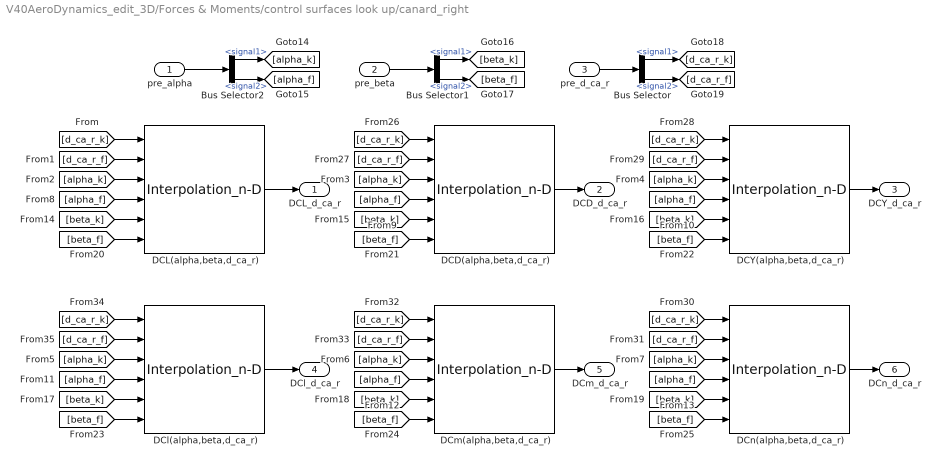
== system V40AeroDynamics_edit_3D/Forces & Moments/control surfaces look up/canard_right ==
  pre_alpha : Inport
  pre_beta : Inport  Port=2
  pre_d_ca_r : Inport  Port=3
  Bus Selector : BusSelector  OutputSignals=signal1,signal2
  Bus Selector1 : BusSelector  OutputSignals=signal1,signal2
  Bus Selector2 : BusSelector  OutputSignals=signal1,signal2
  DCD(alpha,beta,d_ca_r) : Interpolation_n-D  NumberOfTableDimensions=3  Table=CX_d_ca_r{2}  OutDataTypeStr=single
      settings: InputPortMap=u0,u1,u2,u3,u4,u5
  DCL(alpha,beta,d_ca_r) : Interpolation_n-D  NumberOfTableDimensions=3  Table=CX_d_ca_r{1}  OutDataTypeStr=single
      settings: InputPortMap=u0,u1,u2,u3,u4,u5
  DCY(alpha,beta,d_ca_r) : Interpolation_n-D  NumberOfTableDimensions=3  Table=CX_d_ca_r{4}  OutDataTypeStr=single
      settings: InputPortMap=u0,u1,u2,u3,u4,u5
  DCl(alpha,beta,d_ca_r) : Interpolation_n-D  NumberOfTableDimensions=3  Table=CX_d_ca_r{6}  OutDataTypeStr=single
      settings: InputPortMap=u0,u1,u2,u3,u4,u5
  DCm(alpha,beta,d_ca_r) : Interpolation_n-D  NumberOfTableDimensions=3  Table=CX_d_ca_r{3}  OutDataTypeStr=single
      settings: InputPortMap=u0,u1,u2,u3,u4,u5
  DCn(alpha,beta,d_ca_r) : Interpolation_n-D  NumberOfTableDimensions=3  Table=CX_d_ca_r{5}  OutDataTypeStr=single
      settings: InputPortMap=u0,u1,u2,u3,u4,u5
  DCL_d_ca_r : Outport
  DCD_d_ca_r : Outport  Port=2
  DCY_d_ca_r : Outport  Port=3
  DCl_d_ca_r : Outport  Port=4
  DCm_d_ca_r : Outport  Port=5
  DCn_d_ca_r : Outport  Port=6
  wires:
  Bus Selector1/2 -> [beta_f]  "<signal2>"
  DCY(alpha,beta,d_ca_r)/1 -> DCY_d_ca_r/1
  pre_beta/1 -> Bus Selector1/1
  Bus Selector/2 -> [d_ca_r_f]  "<signal2>"
  DCD(alpha,beta,d_ca_r)/1 -> DCD_d_ca_r/1
  DCl(alpha,beta,d_ca_r)/1 -> DCl_d_ca_r/1
  Bus Selector/1 -> [d_ca_r_k]  "<signal1>"
  Bus Selector2/1 -> [alpha_k]  "<signal1>"
  DCm(alpha,beta,d_ca_r)/1 -> DCm_d_ca_r/1
  Bus Selector2/2 -> [alpha_f]  "<signal2>"
  pre_alpha/1 -> Bus Selector2/1
  DCn(alpha,beta,d_ca_r)/1 -> DCn_d_ca_r/1
  DCL(alpha,beta,d_ca_r)/1 -> DCL_d_ca_r/1
  Bus Selector1/1 -> [beta_k]  "<signal1>"
  [d_ca_r_k] -> DCD(alpha,beta,d_ca_r)/1
  [beta_k] -> DCD(alpha,beta,d_ca_r)/5
  [d_ca_r_k] -> DCY(alpha,beta,d_ca_r)/1
  [beta_k] -> DCY(alpha,beta,d_ca_r)/5
  [alpha_k] -> DCY(alpha,beta,d_ca_r)/3
  [d_ca_r_k] -> DCn(alpha,beta,d_ca_r)/1
  [beta_k] -> DCn(alpha,beta,d_ca_r)/5
  [d_ca_r_k] -> DCm(alpha,beta,d_ca_r)/1
  [beta_k] -> DCm(alpha,beta,d_ca_r)/5
  [d_ca_r_k] -> DCL(alpha,beta,d_ca_r)/1
  [d_ca_r_f] -> DCL(alpha,beta,d_ca_r)/2
  [alpha_k] -> DCL(alpha,beta,d_ca_r)/3
  [alpha_f] -> DCL(alpha,beta,d_ca_r)/4
  [beta_k] -> DCL(alpha,beta,d_ca_r)/5
  [beta_f] -> DCL(alpha,beta,d_ca_r)/6
  [d_ca_r_f] -> DCD(alpha,beta,d_ca_r)/2
  [alpha_k] -> DCD(alpha,beta,d_ca_r)/3
  [alpha_f] -> DCD(alpha,beta,d_ca_r)/4
  [beta_f] -> DCD(alpha,beta,d_ca_r)/6
  [d_ca_r_f] -> DCY(alpha,beta,d_ca_r)/2
  [alpha_f] -> DCY(alpha,beta,d_ca_r)/4
  [beta_f] -> DCY(alpha,beta,d_ca_r)/6
  [d_ca_r_f] -> DCn(alpha,beta,d_ca_r)/2
  [alpha_k] -> DCn(alpha,beta,d_ca_r)/3
  [alpha_f] -> DCn(alpha,beta,d_ca_r)/4
  [beta_f] -> DCn(alpha,beta,d_ca_r)/6
  [d_ca_r_f] -> DCm(alpha,beta,d_ca_r)/2
  [alpha_k] -> DCm(alpha,beta,d_ca_r)/3
  [alpha_f] -> DCm(alpha,beta,d_ca_r)/4
  [beta_f] -> DCm(alpha,beta,d_ca_r)/6
  [d_ca_r_k] -> DCl(alpha,beta,d_ca_r)/1
  [d_ca_r_f] -> DCl(alpha,beta,d_ca_r)/2
  [alpha_k] -> DCl(alpha,beta,d_ca_r)/3
  [alpha_f] -> DCl(alpha,beta,d_ca_r)/4
  [beta_k] -> DCl(alpha,beta,d_ca_r)/5
  [beta_f] -> DCl(alpha,beta,d_ca_r)/6
  pre_d_ca_r/1 -> Bus Selector/1

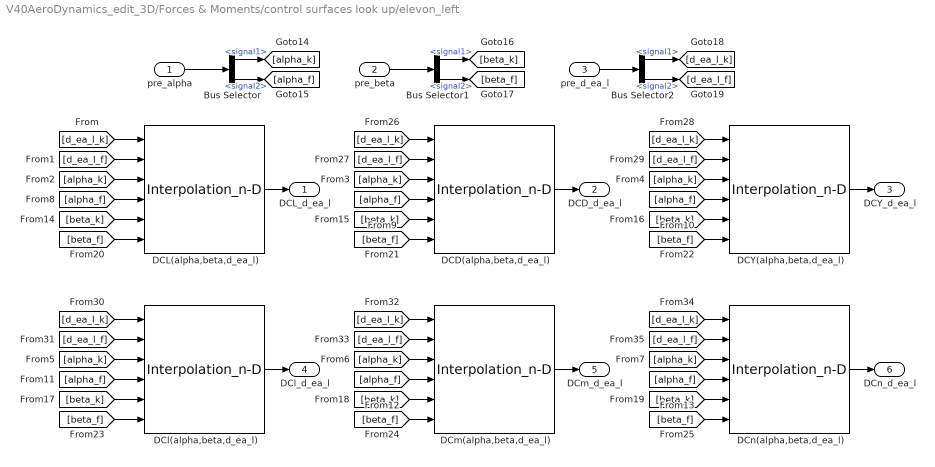
== system V40AeroDynamics_edit_3D/Forces & Moments/control surfaces look up/elevon_left  ==
  pre_alpha : Inport
  pre_beta : Inport  Port=2
  pre_d_ea_l : Inport  Port=3
  Bus Selector : BusSelector  OutputSignals=signal1,signal2
  Bus Selector1 : BusSelector  OutputSignals=signal1,signal2
  Bus Selector2 : BusSelector  OutputSignals=signal1,signal2
  DCD(alpha,beta,d_ea_l) : Interpolation_n-D  NumberOfTableDimensions=3  Table=CX_d_ea_l{2}  OutDataTypeStr=single
      settings: InputPortMap=u0,u1,u2,u3,u4,u5
  DCL(alpha,beta,d_ea_l) : Interpolation_n-D  NumberOfTableDimensions=3  Table=CX_d_ea_l{1}  OutDataTypeStr=single
      settings: InputPortMap=u0,u1,u2,u3,u4,u5
  DCY(alpha,beta,d_ea_l) : Interpolation_n-D  NumberOfTableDimensions=3  Table=CX_d_ea_l{4}  OutDataTypeStr=single
      settings: InputPortMap=u0,u1,u2,u3,u4,u5
  DCl(alpha,beta,d_ea_l) : Interpolation_n-D  NumberOfTableDimensions=3  Table=CX_d_ea_l{6}  OutDataTypeStr=single
      settings: InputPortMap=u0,u1,u2,u3,u4,u5
  DCm(alpha,beta,d_ea_l) : Interpolation_n-D  NumberOfTableDimensions=3  Table=CX_d_ea_l{3}  OutDataTypeStr=single
      settings: InputPortMap=u0,u1,u2,u3,u4,u5
  DCn(alpha,beta,d_ea_l) : Interpolation_n-D  NumberOfTableDimensions=3  Table=CX_d_ea_l{5}  OutDataTypeStr=single
      settings: InputPortMap=u0,u1,u2,u3,u4,u5
  DCL_d_ea_l : Outport
  DCD_d_ea_l : Outport  Port=2
  DCY_d_ea_l : Outport  Port=3
  DCl_d_ea_l : Outport  Port=4
  DCm_d_ea_l : Outport  Port=5
  DCn_d_ea_l : Outport  Port=6
  wires:
  Bus Selector1/2 -> [beta_f]  "<signal2>"
  DCY(alpha,beta,d_ea_l)/1 -> DCY_d_ea_l/1
  pre_beta/1 -> Bus Selector1/1
  Bus Selector2/2 -> [d_ea_l_f]  "<signal2>"
  DCD(alpha,beta,d_ea_l)/1 -> DCD_d_ea_l/1
  DCl(alpha,beta,d_ea_l)/1 -> DCl_d_ea_l/1
  Bus Selector2/1 -> [d_ea_l_k]  "<signal1>"
  Bus Selector/1 -> [alpha_k]  "<signal1>"
  DCm(alpha,beta,d_ea_l)/1 -> DCm_d_ea_l/1
  Bus Selector/2 -> [alpha_f]  "<signal2>"
  pre_alpha/1 -> Bus Selector/1
  DCn(alpha,beta,d_ea_l)/1 -> DCn_d_ea_l/1
  DCL(alpha,beta,d_ea_l)/1 -> DCL_d_ea_l/1
  Bus Selector1/1 -> [beta_k]  "<signal1>"
  [beta_k] -> DCL(alpha,beta,d_ea_l)/5
  [beta_f] -> DCL(alpha,beta,d_ea_l)/6
  [beta_k] -> DCD(alpha,beta,d_ea_l)/5
  [beta_f] -> DCD(alpha,beta,d_ea_l)/6
  [beta_k] -> DCY(alpha,beta,d_ea_l)/5
  [beta_f] -> DCY(alpha,beta,d_ea_l)/6
  [beta_k] -> DCl(alpha,beta,d_ea_l)/5
  [beta_f] -> DCl(alpha,beta,d_ea_l)/6
  [beta_k] -> DCm(alpha,beta,d_ea_l)/5
  [beta_f] -> DCm(alpha,beta,d_ea_l)/6
  [beta_k] -> DCn(alpha,beta,d_ea_l)/5
  [beta_f] -> DCn(alpha,beta,d_ea_l)/6
  [d_ea_l_k] -> DCD(alpha,beta,d_ea_l)/1
  [d_ea_l_k] -> DCY(alpha,beta,d_ea_l)/1
  [d_ea_l_k] -> DCn(alpha,beta,d_ea_l)/1
  [alpha_k] -> DCn(alpha,beta,d_ea_l)/3
  [d_ea_l_k] -> DCm(alpha,beta,d_ea_l)/1
  [alpha_k] -> DCm(alpha,beta,d_ea_l)/3
  [d_ea_l_k] -> DCl(alpha,beta,d_ea_l)/1
  [alpha_k] -> DCl(alpha,beta,d_ea_l)/3
  [d_ea_l_k] -> DCL(alpha,beta,d_ea_l)/1
  [d_ea_l_f] -> DCL(alpha,beta,d_ea_l)/2
  [alpha_k] -> DCL(alpha,beta,d_ea_l)/3
  [alpha_f] -> DCL(alpha,beta,d_ea_l)/4
  [d_ea_l_f] -> DCD(alpha,beta,d_ea_l)/2
  [alpha_k] -> DCD(alpha,beta,d_ea_l)/3
  [alpha_f] -> DCD(alpha,beta,d_ea_l)/4
  [d_ea_l_f] -> DCY(alpha,beta,d_ea_l)/2
  [alpha_k] -> DCY(alpha,beta,d_ea_l)/3
  [alpha_f] -> DCY(alpha,beta,d_ea_l)/4
  [d_ea_l_f] -> DCn(alpha,beta,d_ea_l)/2
  [alpha_f] -> DCn(alpha,beta,d_ea_l)/4
  [d_ea_l_f] -> DCm(alpha,beta,d_ea_l)/2
  [alpha_f] -> DCm(alpha,beta,d_ea_l)/4
  [d_ea_l_f] -> DCl(alpha,beta,d_ea_l)/2
  [alpha_f] -> DCl(alpha,beta,d_ea_l)/4
  pre_d_ea_l/1 -> Bus Selector2/1

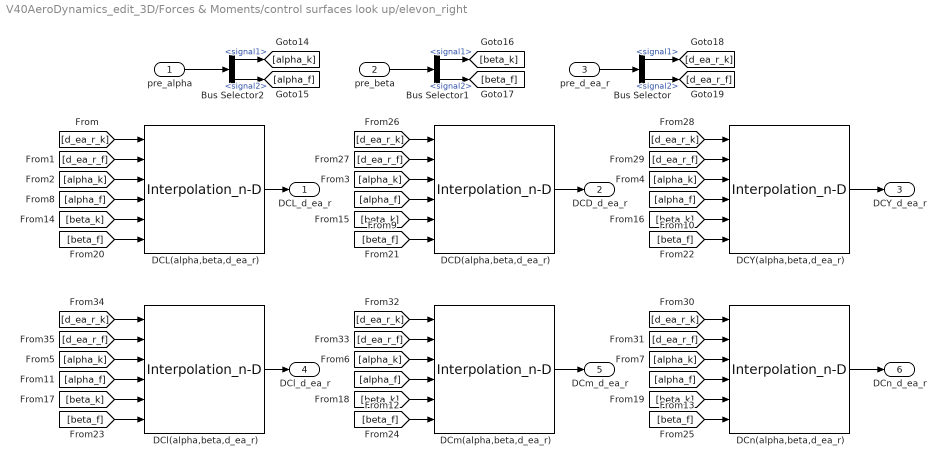
== system V40AeroDynamics_edit_3D/Forces & Moments/control surfaces look up/elevon_right  ==
  pre_alpha : Inport
  pre_beta : Inport  Port=2
  pre_d_ea_r : Inport  Port=3
  Bus Selector : BusSelector  OutputSignals=signal1,signal2
  Bus Selector1 : BusSelector  OutputSignals=signal1,signal2
  Bus Selector2 : BusSelector  OutputSignals=signal1,signal2
  DCD(alpha,beta,d_ea_r) : Interpolation_n-D  NumberOfTableDimensions=3  Table=CX_d_ea_r{2}  OutDataTypeStr=single
      settings: InputPortMap=u0,u1,u2,u3,u4,u5
  DCL(alpha,beta,d_ea_r) : Interpolation_n-D  NumberOfTableDimensions=3  Table=CX_d_ea_r{1}  OutDataTypeStr=single
      settings: InputPortMap=u0,u1,u2,u3,u4,u5
  DCY(alpha,beta,d_ea_r) : Interpolation_n-D  NumberOfTableDimensions=3  Table=CX_d_ea_r{4}  OutDataTypeStr=single
      settings: InputPortMap=u0,u1,u2,u3,u4,u5
  DCl(alpha,beta,d_ea_r) : Interpolation_n-D  NumberOfTableDimensions=3  Table=CX_d_ea_r{6}  OutDataTypeStr=single
      settings: InputPortMap=u0,u1,u2,u3,u4,u5
  DCm(alpha,beta,d_ea_r) : Interpolation_n-D  NumberOfTableDimensions=3  Table=CX_d_ea_r{3}  OutDataTypeStr=single
      settings: InputPortMap=u0,u1,u2,u3,u4,u5
  DCn(alpha,beta,d_ea_r) : Interpolation_n-D  NumberOfTableDimensions=3  Table=CX_d_ea_r{5}  OutDataTypeStr=single
      settings: InputPortMap=u0,u1,u2,u3,u4,u5
  DCL_d_ea_r : Outport
  DCD_d_ea_r : Outport  Port=2
  DCY_d_ea_r : Outport  Port=3
  DCl_d_ea_r : Outport  Port=4
  DCm_d_ea_r : Outport  Port=5
  DCn_d_ea_r : Outport  Port=6
  wires:
  Bus Selector1/2 -> [beta_f]  "<signal2>"
  DCY(alpha,beta,d_ea_r)/1 -> DCY_d_ea_r/1
  pre_beta/1 -> Bus Selector1/1
  Bus Selector/2 -> [d_ea_r_f]  "<signal2>"
  DCD(alpha,beta,d_ea_r)/1 -> DCD_d_ea_r/1
  DCl(alpha,beta,d_ea_r)/1 -> DCl_d_ea_r/1
  Bus Selector/1 -> [d_ea_r_k]  "<signal1>"
  Bus Selector2/1 -> [alpha_k]  "<signal1>"
  DCm(alpha,beta,d_ea_r)/1 -> DCm_d_ea_r/1
  Bus Selector2/2 -> [alpha_f]  "<signal2>"
  pre_alpha/1 -> Bus Selector2/1
  DCn(alpha,beta,d_ea_r)/1 -> DCn_d_ea_r/1
  DCL(alpha,beta,d_ea_r)/1 -> DCL_d_ea_r/1
  Bus Selector1/1 -> [beta_k]  "<signal1>"
  [beta_k] -> DCL(alpha,beta,d_ea_r)/5
  [beta_f] -> DCL(alpha,beta,d_ea_r)/6
  [beta_k] -> DCD(alpha,beta,d_ea_r)/5
  [beta_f] -> DCD(alpha,beta,d_ea_r)/6
  [beta_k] -> DCY(alpha,beta,d_ea_r)/5
  [beta_f] -> DCY(alpha,beta,d_ea_r)/6
  [beta_k] -> DCl(alpha,beta,d_ea_r)/5
  [beta_f] -> DCl(alpha,beta,d_ea_r)/6
  [beta_k] -> DCm(alpha,beta,d_ea_r)/5
  [beta_f] -> DCm(alpha,beta,d_ea_r)/6
  [beta_k] -> DCn(alpha,beta,d_ea_r)/5
  [beta_f] -> DCn(alpha,beta,d_ea_r)/6
  [d_ea_r_k] -> DCD(alpha,beta,d_ea_r)/1
  [d_ea_r_k] -> DCY(alpha,beta,d_ea_r)/1
  [d_ea_r_k] -> DCn(alpha,beta,d_ea_r)/1
  [d_ea_r_k] -> DCm(alpha,beta,d_ea_r)/1
  [d_ea_r_k] -> DCL(alpha,beta,d_ea_r)/1
  [d_ea_r_f] -> DCL(alpha,beta,d_ea_r)/2
  [alpha_k] -> DCL(alpha,beta,d_ea_r)/3
  [alpha_f] -> DCL(alpha,beta,d_ea_r)/4
  [d_ea_r_f] -> DCD(alpha,beta,d_ea_r)/2
  [alpha_k] -> DCD(alpha,beta,d_ea_r)/3
  [alpha_f] -> DCD(alpha,beta,d_ea_r)/4
  [d_ea_r_f] -> DCY(alpha,beta,d_ea_r)/2
  [alpha_k] -> DCY(alpha,beta,d_ea_r)/3
  [alpha_f] -> DCY(alpha,beta,d_ea_r)/4
  [d_ea_r_f] -> DCn(alpha,beta,d_ea_r)/2
  [alpha_k] -> DCn(alpha,beta,d_ea_r)/3
  [alpha_f] -> DCn(alpha,beta,d_ea_r)/4
  [d_ea_r_f] -> DCm(alpha,beta,d_ea_r)/2
  [alpha_k] -> DCm(alpha,beta,d_ea_r)/3
  [alpha_f] -> DCm(alpha,beta,d_ea_r)/4
  [d_ea_r_k] -> DCl(alpha,beta,d_ea_r)/1
  [d_ea_r_f] -> DCl(alpha,beta,d_ea_r)/2
  [alpha_k] -> DCl(alpha,beta,d_ea_r)/3
  [alpha_f] -> DCl(alpha,beta,d_ea_r)/4
  pre_d_ea_r/1 -> Bus Selector/1

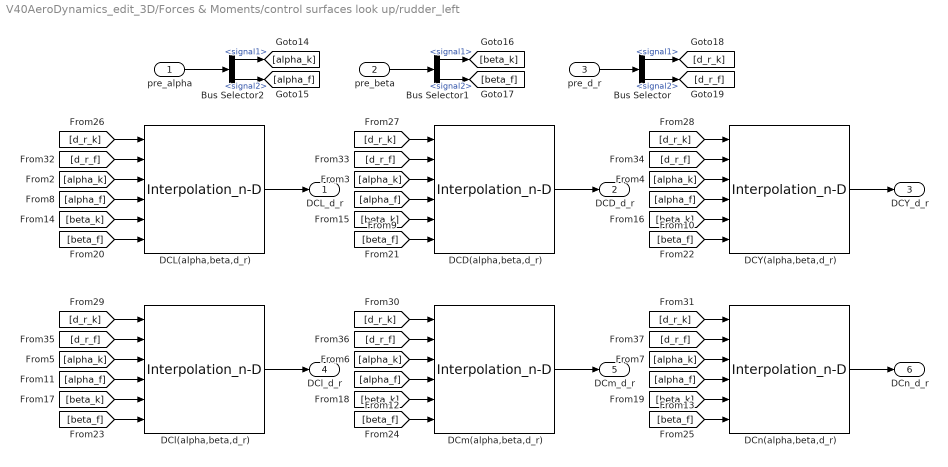
== system V40AeroDynamics_edit_3D/Forces & Moments/control surfaces look up/rudder_left ==
  pre_alpha : Inport
  pre_beta : Inport  Port=2
  pre_d_r : Inport  Port=3
  Bus Selector : BusSelector  OutputSignals=signal1,signal2
  Bus Selector1 : BusSelector  OutputSignals=signal1,signal2
  Bus Selector2 : BusSelector  OutputSignals=signal1,signal2
  DCD(alpha,beta,d_r) : Interpolation_n-D  NumberOfTableDimensions=3  Table=CX_d_r{2}  OutDataTypeStr=single
      settings: InputPortMap=u0,u1,u2,u3,u4,u5
  DCL(alpha,beta,d_r) : Interpolation_n-D  NumberOfTableDimensions=3  Table=CX_d_r{1}  OutDataTypeStr=single
      settings: InputPortMap=u0,u1,u2,u3,u4,u5
  DCY(alpha,beta,d_r) : Interpolation_n-D  NumberOfTableDimensions=3  Table=CX_d_r{4}  OutDataTypeStr=single
      settings: InputPortMap=u0,u1,u2,u3,u4,u5
  DCl(alpha,beta,d_r) : Interpolation_n-D  NumberOfTableDimensions=3  Table=CX_d_r{6}  OutDataTypeStr=single
      settings: InputPortMap=u0,u1,u2,u3,u4,u5
  DCm(alpha,beta,d_r) : Interpolation_n-D  NumberOfTableDimensions=3  Table=CX_d_r{3}  OutDataTypeStr=single
      settings: InputPortMap=u0,u1,u2,u3,u4,u5
  DCn(alpha,beta,d_r) : Interpolation_n-D  NumberOfTableDimensions=3  Table=CX_d_r{5}  OutDataTypeStr=single
      settings: InputPortMap=u0,u1,u2,u3,u4,u5
  DCL_d_r : Outport
  DCD_d_r : Outport  Port=2
  DCY_d_r : Outport  Port=3
  DCl_d_r : Outport  Port=4
  DCm_d_r : Outport  Port=5
  DCn_d_r : Outport  Port=6
  wires:
  Bus Selector1/2 -> [beta_f]  "<signal2>"
  DCY(alpha,beta,d_r)/1 -> DCY_d_r/1
  pre_beta/1 -> Bus Selector1/1
  Bus Selector/2 -> [d_r_f]  "<signal2>"
  DCD(alpha,beta,d_r)/1 -> DCD_d_r/1
  DCl(alpha,beta,d_r)/1 -> DCl_d_r/1
  Bus Selector/1 -> [d_r_k]  "<signal1>"
  Bus Selector2/1 -> [alpha_k]  "<signal1>"
  DCm(alpha,beta,d_r)/1 -> DCm_d_r/1
  Bus Selector2/2 -> [alpha_f]  "<signal2>"
  pre_alpha/1 -> Bus Selector2/1
  DCn(alpha,beta,d_r)/1 -> DCn_d_r/1
  DCL(alpha,beta,d_r)/1 -> DCL_d_r/1
  Bus Selector1/1 -> [beta_k]  "<signal1>"
  [d_r_k] -> DCD(alpha,beta,d_r)/1
  [beta_k] -> DCD(alpha,beta,d_r)/5
  [d_r_k] -> DCY(alpha,beta,d_r)/1
  [beta_k] -> DCY(alpha,beta,d_r)/5
  [alpha_k] -> DCY(alpha,beta,d_r)/3
  [d_r_k] -> DCn(alpha,beta,d_r)/1
  [beta_k] -> DCn(alpha,beta,d_r)/5
  [d_r_k] -> DCm(alpha,beta,d_r)/1
  [beta_k] -> DCm(alpha,beta,d_r)/5
  [d_r_k] -> DCL(alpha,beta,d_r)/1
  [d_r_f] -> DCL(alpha,beta,d_r)/2
  [alpha_k] -> DCL(alpha,beta,d_r)/3
  [alpha_f] -> DCL(alpha,beta,d_r)/4
  [beta_k] -> DCL(alpha,beta,d_r)/5
  [beta_f] -> DCL(alpha,beta,d_r)/6
  [d_r_f] -> DCD(alpha,beta,d_r)/2
  [alpha_k] -> DCD(alpha,beta,d_r)/3
  [alpha_f] -> DCD(alpha,beta,d_r)/4
  [beta_f] -> DCD(alpha,beta,d_r)/6
  [d_r_f] -> DCY(alpha,beta,d_r)/2
  [alpha_f] -> DCY(alpha,beta,d_r)/4
  [beta_f] -> DCY(alpha,beta,d_r)/6
  [d_r_f] -> DCn(alpha,beta,d_r)/2
  [alpha_k] -> DCn(alpha,beta,d_r)/3
  [alpha_f] -> DCn(alpha,beta,d_r)/4
  [beta_f] -> DCn(alpha,beta,d_r)/6
  [d_r_f] -> DCm(alpha,beta,d_r)/2
  [alpha_k] -> DCm(alpha,beta,d_r)/3
  [alpha_f] -> DCm(alpha,beta,d_r)/4
  [beta_f] -> DCm(alpha,beta,d_r)/6
  [d_r_k] -> DCl(alpha,beta,d_r)/1
  [d_r_f] -> DCl(alpha,beta,d_r)/2
  [alpha_k] -> DCl(alpha,beta,d_r)/3
  [alpha_f] -> DCl(alpha,beta,d_r)/4
  [beta_k] -> DCl(alpha,beta,d_r)/5
  [beta_f] -> DCl(alpha,beta,d_r)/6
  pre_d_r/1 -> Bus Selector/1

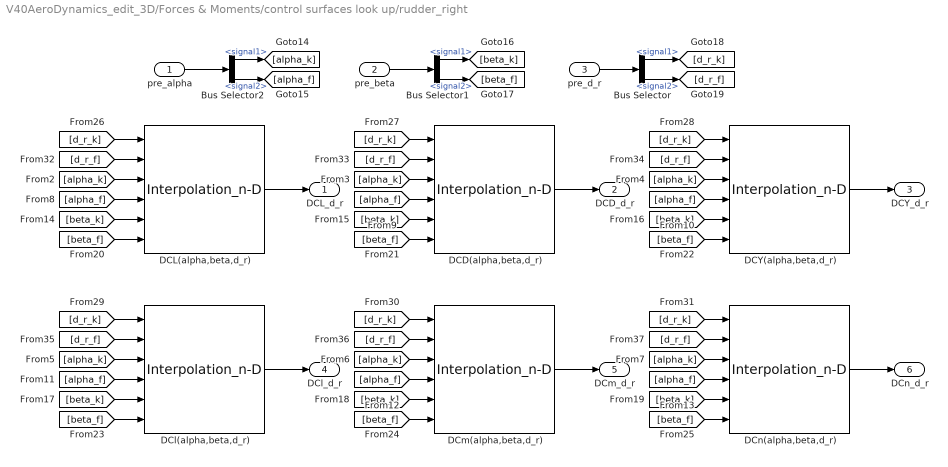
== system V40AeroDynamics_edit_3D/Forces & Moments/control surfaces look up/rudder_right ==
  pre_alpha : Inport
  pre_beta : Inport  Port=2
  pre_d_r : Inport  Port=3
  Bus Selector : BusSelector  OutputSignals=signal1,signal2
  Bus Selector1 : BusSelector  OutputSignals=signal1,signal2
  Bus Selector2 : BusSelector  OutputSignals=signal1,signal2
  DCD(alpha,beta,d_r) : Interpolation_n-D  NumberOfTableDimensions=3  Table=CX_d_r{2}  OutDataTypeStr=single
      settings: InputPortMap=u0,u1,u2,u3,u4,u5
  DCL(alpha,beta,d_r) : Interpolation_n-D  NumberOfTableDimensions=3  Table=CX_d_r{1}  OutDataTypeStr=single
      settings: InputPortMap=u0,u1,u2,u3,u4,u5
  DCY(alpha,beta,d_r) : Interpolation_n-D  NumberOfTableDimensions=3  Table=CX_d_r{4}  OutDataTypeStr=single
      settings: InputPortMap=u0,u1,u2,u3,u4,u5
  DCl(alpha,beta,d_r) : Interpolation_n-D  NumberOfTableDimensions=3  Table=CX_d_r{6}  OutDataTypeStr=single
      settings: InputPortMap=u0,u1,u2,u3,u4,u5
  DCm(alpha,beta,d_r) : Interpolation_n-D  NumberOfTableDimensions=3  Table=CX_d_r{3}  OutDataTypeStr=single
      settings: InputPortMap=u0,u1,u2,u3,u4,u5
  DCn(alpha,beta,d_r) : Interpolation_n-D  NumberOfTableDimensions=3  Table=CX_d_r{5}  OutDataTypeStr=single
      settings: InputPortMap=u0,u1,u2,u3,u4,u5
  DCL_d_r : Outport
  DCD_d_r : Outport  Port=2
  DCY_d_r : Outport  Port=3
  DCl_d_r : Outport  Port=4
  DCm_d_r : Outport  Port=5
  DCn_d_r : Outport  Port=6
  wires:
  Bus Selector1/2 -> [beta_f]  "<signal2>"
  DCY(alpha,beta,d_r)/1 -> DCY_d_r/1
  pre_beta/1 -> Bus Selector1/1
  Bus Selector/2 -> [d_r_f]  "<signal2>"
  DCD(alpha,beta,d_r)/1 -> DCD_d_r/1
  DCl(alpha,beta,d_r)/1 -> DCl_d_r/1
  Bus Selector/1 -> [d_r_k]  "<signal1>"
  Bus Selector2/1 -> [alpha_k]  "<signal1>"
  DCm(alpha,beta,d_r)/1 -> DCm_d_r/1
  Bus Selector2/2 -> [alpha_f]  "<signal2>"
  pre_alpha/1 -> Bus Selector2/1
  DCn(alpha,beta,d_r)/1 -> DCn_d_r/1
  DCL(alpha,beta,d_r)/1 -> DCL_d_r/1
  Bus Selector1/1 -> [beta_k]  "<signal1>"
  [d_r_k] -> DCD(alpha,beta,d_r)/1
  [beta_k] -> DCD(alpha,beta,d_r)/5
  [d_r_k] -> DCY(alpha,beta,d_r)/1
  [beta_k] -> DCY(alpha,beta,d_r)/5
  [alpha_k] -> DCY(alpha,beta,d_r)/3
  [d_r_k] -> DCn(alpha,beta,d_r)/1
  [beta_k] -> DCn(alpha,beta,d_r)/5
  [d_r_k] -> DCm(alpha,beta,d_r)/1
  [beta_k] -> DCm(alpha,beta,d_r)/5
  [d_r_k] -> DCL(alpha,beta,d_r)/1
  [d_r_f] -> DCL(alpha,beta,d_r)/2
  [alpha_k] -> DCL(alpha,beta,d_r)/3
  [alpha_f] -> DCL(alpha,beta,d_r)/4
  [beta_k] -> DCL(alpha,beta,d_r)/5
  [beta_f] -> DCL(alpha,beta,d_r)/6
  [d_r_f] -> DCD(alpha,beta,d_r)/2
  [alpha_k] -> DCD(alpha,beta,d_r)/3
  [alpha_f] -> DCD(alpha,beta,d_r)/4
  [beta_f] -> DCD(alpha,beta,d_r)/6
  [d_r_f] -> DCY(alpha,beta,d_r)/2
  [alpha_f] -> DCY(alpha,beta,d_r)/4
  [beta_f] -> DCY(alpha,beta,d_r)/6
  [d_r_f] -> DCn(alpha,beta,d_r)/2
  [alpha_k] -> DCn(alpha,beta,d_r)/3
  [alpha_f] -> DCn(alpha,beta,d_r)/4
  [beta_f] -> DCn(alpha,beta,d_r)/6
  [d_r_f] -> DCm(alpha,beta,d_r)/2
  [alpha_k] -> DCm(alpha,beta,d_r)/3
  [alpha_f] -> DCm(alpha,beta,d_r)/4
  [beta_f] -> DCm(alpha,beta,d_r)/6
  [d_r_k] -> DCl(alpha,beta,d_r)/1
  [d_r_f] -> DCl(alpha,beta,d_r)/2
  [alpha_k] -> DCl(alpha,beta,d_r)/3
  [alpha_f] -> DCl(alpha,beta,d_r)/4
  [beta_k] -> DCl(alpha,beta,d_r)/5
  [beta_f] -> DCl(alpha,beta,d_r)/6
  pre_d_r/1 -> Bus Selector/1

== system V40AeroDynamics_edit_3D/Forces & Moments/summation/coef computation ==
  In : Inport
  Add1 : Sum  Inputs=+++++++++
  Demux : Demux  Outputs=9
  Out : Outport
  wires:
  In/1 -> Demux/1
  Add1/1 -> Out/1
  Demux/1 -> Add1/1
  Demux/9 -> Add1/9
  Demux/8 -> Add1/8
  Demux/7 -> Add1/7
  Demux/6 -> Add1/6
  Demux/5 -> Add1/5
  Demux/4 -> Add1/4
  Demux/2 -> Add1/2
  Demux/3 -> Add1/3

== system V40AeroDynamics_edit_3D/Forces & Moments/summation/coef computation1 ==
  In : Inport
  Add1 : Sum  Inputs=++++++++
  Demux : Demux  Outputs=8
  Out : Outport
  wires:
  In/1 -> Demux/1
  Add1/1 -> Out/1
  Demux/1 -> Add1/1
  Demux/2 -> Add1/2
  Demux/3 -> Add1/3
  Demux/4 -> Add1/4
  Demux/5 -> Add1/5
  Demux/6 -> Add1/6
  Demux/7 -> Add1/7
  Demux/8 -> Add1/8

== system V40AeroDynamics_edit_3D/Forces & Moments/summation/coef computation2 ==
  In : Inport
  Add1 : Sum  Inputs=+++++++
  Demux : Demux  Outputs=7
  Out : Outport
  wires:
  In/1 -> Demux/1
  Add1/1 -> Out/1
  Demux/1 -> Add1/1
  Demux/2 -> Add1/2
  Demux/3 -> Add1/3
  Demux/4 -> Add1/4
  Demux/5 -> Add1/5
  Demux/6 -> Add1/6
  Demux/7 -> Add1/7
